simulink model "holidays11"  (R2019a)
settings: Solver=VariableStepAuto  StartTime=0.0  StopTime=5.0  RelTol=1e-3
libraries: dspsigops x1, dspmathops x1
settings Model: Creator=Aditya  LastModifiedBy=Aditya

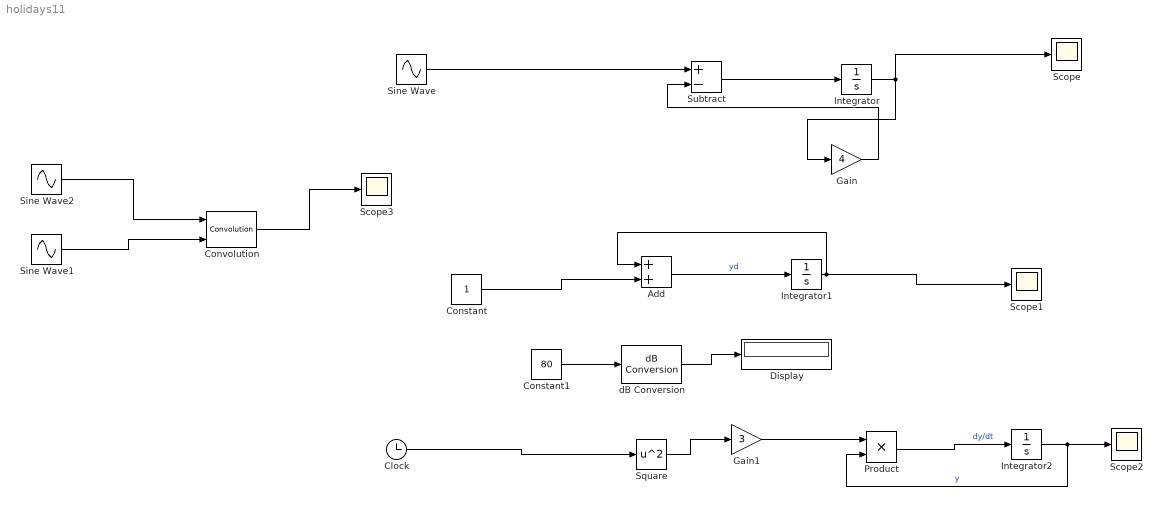
== system holidays11 ==
  Add : Sum
  Clock : Clock
  Constant : Constant
  Constant1 : Constant  Value=80
  Convolution : dspsigops/Convolution  domain=Time  roundingMode=Floor  overflowMode=off  outputDataTypeStr=Inherit: Same as accumulator  outputMin=[]  outputMax=[]  outputLastDataTypeStr=Inherit: Same as accumulator
      settings: SourceProductName=DSP System Toolbox  SourceProductBaseCode=DS
  Display : Display
  Gain : Gain  Gain=4
  Gain1 : Gain  Gain=3
  Integrator : Integrator
  Integrator1 : Integrator
  Integrator2 : Integrator  InitialCondition=1
  Product : Product
  Scope{,1..3} (4 alike) : Scope
  Sine Wave : Sin  Amplitude=2  Frequency=3  SampleTime=0
  Sine Wave1 : Sin  SampleTime=0
  Sine Wave2 : Sin  SampleTime=0
  Square : Math  Operator=square  SaturateOnIntegerOverflow=on
  Subtract : Sum  Inputs=+-
  dB Conversion : dspmathops/dB Conversion  dBtype=dB  intype=Amplitude  R=1  fuzz=off
      settings: SourceProductName=DSP System Toolbox
  wires:
  Sine Wave/1 -> Subtract/1
  Subtract/1 -> Integrator/1
  Integrator/1 -> Scope/1, Gain/1
  Gain/1 -> Subtract/2
  Add/1 -> Integrator1/1  "yd"
  Integrator1/1 -> Add/1, Scope1/1
  Constant/1 -> Add/2
  Clock/1 -> Square/1
  Square/1 -> Gain1/1
  Gain1/1 -> Product/1
  Product/1 -> Integrator2/1  "dy/dt"
  Integrator2/1 -> Product/2, Scope2/1  "y"
  Constant1/1 -> dB Conversion/1
  dB Conversion/1 -> Display/1
  Sine Wave1/1 -> Convolution/2
  Sine Wave2/1 -> Convolution/1
  Convolution/1 -> Scope3/1
